simulink model "gearbox"  (R2019b)
settings: Solver=VariableStepAuto  StartTime=0.0  StopTime=10.0  RelTol=1e-3
settings Model: Creator=Avmash  LastModifiedBy=Avmash

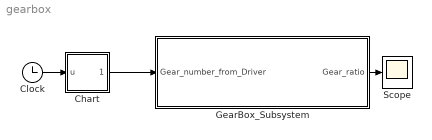
== system gearbox ==
  Chart : Stateflow chart  BlockKeywords=__PRM__SERIALIZED__DATA__:Stateflow Chart,Stateflow Diagram  TreatAsAtomicUnit=on
  Clock : Clock
  GearBox_Subsystem : Subsystem
  Scope : Scope
  wires:
  Clock/1 -> Chart/1(u)
  GearBox_Subsystem/1(Gear_ratio) -> Scope/1
  Chart/1(Gear) -> GearBox_Subsystem/1(Gear_number_from_Driver)

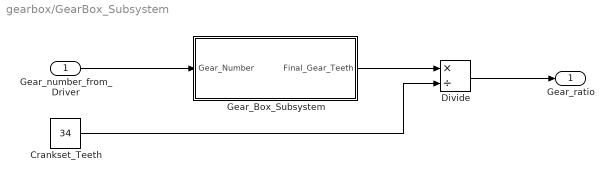
== system gearbox/GearBox_Subsystem ==
  Gear_number_from_Driver : Inport
  Crankset_Teeth : Constant  Value=34
  Divide : Product  Inputs=*/
  Gear_Box_Subsystem : Subsystem
  Gear_ratio : Outport  VectorParamsAs1DForOutWhenUnconnected=off
  wires:
  Divide/1 -> Gear_ratio/1
  Gear_number_from_Driver/1 -> Gear_Box_Subsystem/1(Gear_Number)
  Gear_Box_Subsystem/1(Final_Gear_Teeth) -> Divide/1
  Crankset_Teeth/1 -> Divide/2

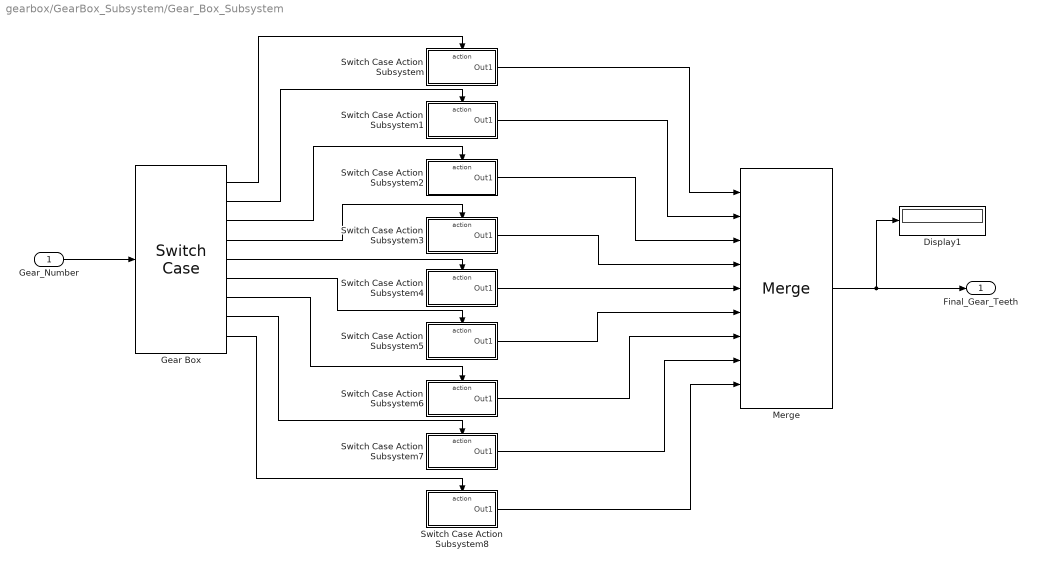
== system gearbox/GearBox_Subsystem/Gear_Box_Subsystem ==
  Gear_Number : Inport
  Display1 : Display
  Gear Box : SwitchCase  CaseConditions={1,2,3,4,5,6,7,8,9}  ShowDefaultCase=off
  Merge : Merge  Inputs=9
  Switch Case Action Subsystem : Subsystem  TreatAsAtomicUnit=on
  Switch Case Action Subsystem1 : Subsystem  TreatAsAtomicUnit=on
  Switch Case Action Subsystem2 : Subsystem  TreatAsAtomicUnit=on
  Switch Case Action Subsystem3 : Subsystem  TreatAsAtomicUnit=on
  Switch Case Action Subsystem4 : Subsystem  TreatAsAtomicUnit=on
  Switch Case Action Subsystem5 : Subsystem  TreatAsAtomicUnit=on
  Switch Case Action Subsystem6 : Subsystem  TreatAsAtomicUnit=on
  Switch Case Action Subsystem7 : Subsystem  TreatAsAtomicUnit=on
  Switch Case Action Subsystem8 : Subsystem  TreatAsAtomicUnit=on
  Final_Gear_Teeth : Outport  VectorParamsAs1DForOutWhenUnconnected=off
  wires:
  Gear Box/5 -> Switch Case Action Subsystem4/Action
  Gear Box/2 -> Switch Case Action Subsystem1/Action
  Gear Box/4 -> Switch Case Action Subsystem3/Action
  Gear Box/9 -> Switch Case Action Subsystem8/Action
  Gear Box/7 -> Switch Case Action Subsystem6/Action
  Gear Box/6 -> Switch Case Action Subsystem5/Action
  Gear Box/3 -> Switch Case Action Subsystem2/Action
  Gear Box/1 -> Switch Case Action Subsystem/Action
  Merge/1 -> Display1/1, Final_Gear_Teeth/1
  Gear Box/8 -> Switch Case Action Subsystem7/Action
  Gear_Number/1 -> Gear Box/1
  Switch Case Action Subsystem8/1(Out1) -> Merge/9
  Switch Case Action Subsystem7/1(Out1) -> Merge/8
  Switch Case Action Subsystem6/1(Out1) -> Merge/7
  Switch Case Action Subsystem5/1(Out1) -> Merge/6
  Switch Case Action Subsystem4/1(Out1) -> Merge/5
  Switch Case Action Subsystem3/1(Out1) -> Merge/4
  Switch Case Action Subsystem2/1(Out1) -> Merge/3
  Switch Case Action Subsystem1/1(Out1) -> Merge/2
  Switch Case Action Subsystem/1(Out1) -> Merge/1

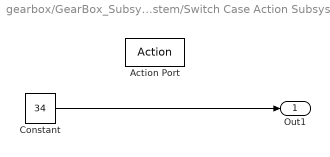
== system gearbox/GearBox_Subsystem/Gear_Box_Subsystem/Switch Case Action Subsystem ==
  Action Port : ActionPort  ActionPortLabel=case [ 1 ]:
  Constant : Constant  Value=34
  Out1 : Outport  VectorParamsAs1DForOutWhenUnconnected=off
  wires:
  Constant/1 -> Out1/1

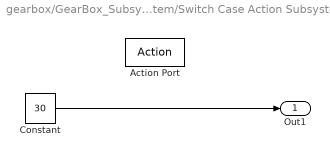
== system gearbox/GearBox_Subsystem/Gear_Box_Subsystem/Switch Case Action Subsystem1 ==
  Action Port : ActionPort  ActionPortLabel=case [ 2 ]:
  Constant : Constant  Value=30
  Out1 : Outport  VectorParamsAs1DForOutWhenUnconnected=off
  wires:
  Constant/1 -> Out1/1

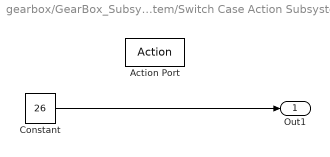
== system gearbox/GearBox_Subsystem/Gear_Box_Subsystem/Switch Case Action Subsystem2 ==
  Action Port : ActionPort  ActionPortLabel=case [ 3 ]:
  Constant : Constant  Value=26
  Out1 : Outport  VectorParamsAs1DForOutWhenUnconnected=off
  wires:
  Constant/1 -> Out1/1

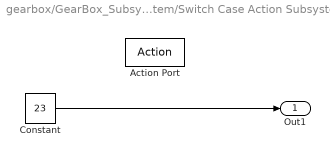
== system gearbox/GearBox_Subsystem/Gear_Box_Subsystem/Switch Case Action Subsystem3 ==
  Action Port : ActionPort  ActionPortLabel=case [ 4 ]:
  Constant : Constant  Value=23
  Out1 : Outport  VectorParamsAs1DForOutWhenUnconnected=off
  wires:
  Constant/1 -> Out1/1

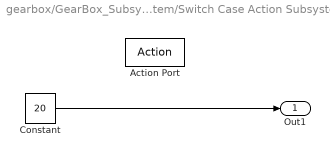
== system gearbox/GearBox_Subsystem/Gear_Box_Subsystem/Switch Case Action Subsystem4 ==
  Action Port : ActionPort  ActionPortLabel=case [ 5 ]:
  Constant : Constant  Value=20
  Out1 : Outport  VectorParamsAs1DForOutWhenUnconnected=off
  wires:
  Constant/1 -> Out1/1

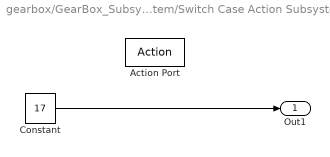
== system gearbox/GearBox_Subsystem/Gear_Box_Subsystem/Switch Case Action Subsystem5 ==
  Action Port : ActionPort  ActionPortLabel=case [ 6 ]:
  Constant : Constant  Value=17
  Out1 : Outport  VectorParamsAs1DForOutWhenUnconnected=off
  wires:
  Constant/1 -> Out1/1

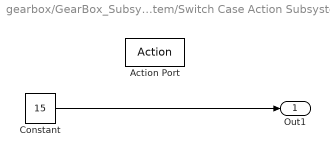
== system gearbox/GearBox_Subsystem/Gear_Box_Subsystem/Switch Case Action Subsystem6 ==
  Action Port : ActionPort  ActionPortLabel=case [ 7 ]:
  Constant : Constant  Value=15
  Out1 : Outport  VectorParamsAs1DForOutWhenUnconnected=off
  wires:
  Constant/1 -> Out1/1

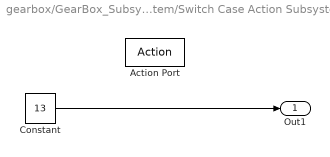
== system gearbox/GearBox_Subsystem/Gear_Box_Subsystem/Switch Case Action Subsystem7 ==
  Action Port : ActionPort  ActionPortLabel=case [ 8 ]:
  Constant : Constant  Value=13
  Out1 : Outport  VectorParamsAs1DForOutWhenUnconnected=off
  wires:
  Constant/1 -> Out1/1

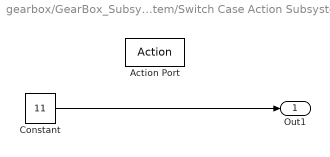
== system gearbox/GearBox_Subsystem/Gear_Box_Subsystem/Switch Case Action Subsystem8 ==
  Action Port : ActionPort  ActionPortLabel=case [ 9 ]:
  Constant : Constant  Value=11
  Out1 : Outport  VectorParamsAs1DForOutWhenUnconnected=off
  wires:
  Constant/1 -> Out1/1

== stateflow chart gearbox/Chart ==
  (junction 5) -> (junction 9) : {Gear=1}
  (junction 2) -> (junction 5) [order 1] : [u==0&& u<1]
  (junction 9) -> (junction 15)
  (junction 7) -> (junction 13) : {Gear=2}
  (junction 2) -> (junction 7) [order 2] : [u==1&& u<2]
  (junction 13) -> (junction 15)
  (junction 25) -> (junction 28) : {Gear=3}
  (junction 2) -> (junction 25) [order 3] : [u==2&& u<3]
  (junction 28) -> (junction 15)
  (junction 36) -> (junction 34) : {Gear=4}
  (junction 2) -> (junction 36) [order 4] : [u==3&& u<4]
  (junction 34) -> (junction 15)
  (default) -> (junction 2)
  (junction 2) -> (junction 41) [order 5] : [u==4&& u<5]
  (junction 41) -> (junction 38) : {Gear=5}
  (junction 38) -> (junction 15)
  (junction 15) -> (junction 18)
  (junction 2) -> (junction 42) [order 6] : [u==5&& u<6]
  (junction 43) -> (junction 15)
  (junction 2) -> (junction 51) [order 7] : [u==6&& u<7]
  (junction 48) -> (junction 15)
  (junction 2) -> (junction 57) [order 8] : [u==7&& u<8]
  (junction 2) -> (junction 74) [order 9] : [u==8&& u<9]
  (junction 59) -> (junction 15)
  (junction 76) -> (junction 15)
  (junction 42) -> (junction 43) : {Gear=6}
  (junction 51) -> (junction 48) : {Gear=7}
  (junction 57) -> (junction 59) : {Gear=8}
  (junction 74) -> (junction 76) : {Gear=9}
  data: u input; Gear output
